simulink model "UZ_EnDat_be4_optimizing_agaib"  (R2023b)
settings: Solver=FixedStepDiscrete  StartTime=0  StopTime=0.002  RelTol=1e-3
model workspace (MAT data in the model file):
  Select = 0
libraries: hdlsllib x750, simulink x19, simulink_extras x4
(part 7 of 9)

== system UZ_EnDat_be4_optimizing_agaib/UZ_ENDAT/ManualSerialize/padder/nibblepadding22/padding1 ==
  in : Inport
  Bit Shift2 : hdlsllib/Logic and Bit Operations/Bit Shift  mode=Shift Right Logical  N=1
  Bit Slice2 : hdlsllib/Logic and Bit Operations/Bit Slice  lidx=0  ridx=0
  Data Type Conversion2 : DataTypeConversion  OutDataTypeStr=boolean  RndMeth=Nearest  SaturateOnIntegerOverflow=off
  Switch2 : Switch  Criteria=u2 > Threshold  SaturateOnIntegerOverflow=off  InputSameDT=off
  out : Outport
  wires:
  in/1 -> Bit Shift2/1, Switch2/1, Bit Slice2/1
  Bit Shift2/1 -> Switch2/3
  Data Type Conversion2/1 -> Switch2/2
  Bit Slice2/1 -> Data Type Conversion2/1
  Switch2/1 -> out/1

== system UZ_EnDat_be4_optimizing_agaib/UZ_ENDAT/ManualSerialize/padder/nibblepadding22/padding2 ==
  in : Inport
  Bit Shift2 : hdlsllib/Logic and Bit Operations/Bit Shift  mode=Shift Right Logical  N=1
  Bit Slice2 : hdlsllib/Logic and Bit Operations/Bit Slice  lidx=0  ridx=0
  Data Type Conversion2 : DataTypeConversion  OutDataTypeStr=boolean  RndMeth=Nearest  SaturateOnIntegerOverflow=off
  Switch2 : Switch  Criteria=u2 > Threshold  SaturateOnIntegerOverflow=off  InputSameDT=off
  out : Outport
  wires:
  in/1 -> Bit Shift2/1, Switch2/1, Bit Slice2/1
  Bit Shift2/1 -> Switch2/3
  Data Type Conversion2/1 -> Switch2/2
  Bit Slice2/1 -> Data Type Conversion2/1
  Switch2/1 -> out/1

== system UZ_EnDat_be4_optimizing_agaib/UZ_ENDAT/ManualSerialize/padder/nibblepadding22/padding3 ==
  in : Inport
  Bit Shift2 : hdlsllib/Logic and Bit Operations/Bit Shift  mode=Shift Right Logical  N=1
  Bit Slice2 : hdlsllib/Logic and Bit Operations/Bit Slice  lidx=0  ridx=0
  Data Type Conversion2 : DataTypeConversion  OutDataTypeStr=boolean  RndMeth=Nearest  SaturateOnIntegerOverflow=off
  Switch2 : Switch  Criteria=u2 > Threshold  SaturateOnIntegerOverflow=off  InputSameDT=off
  out : Outport
  wires:
  in/1 -> Bit Shift2/1, Switch2/1, Bit Slice2/1
  Bit Shift2/1 -> Switch2/3
  Data Type Conversion2/1 -> Switch2/2
  Bit Slice2/1 -> Data Type Conversion2/1
  Switch2/1 -> out/1

== system UZ_EnDat_be4_optimizing_agaib/UZ_ENDAT/ManualSerialize/padder/nibblepadding23/padding ==
  in : Inport
  Bit Shift2 : hdlsllib/Logic and Bit Operations/Bit Shift  mode=Shift Right Logical  N=1
  Bit Slice2 : hdlsllib/Logic and Bit Operations/Bit Slice  lidx=0  ridx=0
  Data Type Conversion2 : DataTypeConversion  OutDataTypeStr=boolean  RndMeth=Nearest  SaturateOnIntegerOverflow=off
  Switch2 : Switch  Criteria=u2 > Threshold  SaturateOnIntegerOverflow=off  InputSameDT=off
  out : Outport
  wires:
  in/1 -> Bit Shift2/1, Switch2/1, Bit Slice2/1
  Bit Shift2/1 -> Switch2/3
  Data Type Conversion2/1 -> Switch2/2
  Bit Slice2/1 -> Data Type Conversion2/1
  Switch2/1 -> out/1

== system UZ_EnDat_be4_optimizing_agaib/UZ_ENDAT/ManualSerialize/padder/nibblepadding23/padding1 ==
  in : Inport
  Bit Shift2 : hdlsllib/Logic and Bit Operations/Bit Shift  mode=Shift Right Logical  N=1
  Bit Slice2 : hdlsllib/Logic and Bit Operations/Bit Slice  lidx=0  ridx=0
  Data Type Conversion2 : DataTypeConversion  OutDataTypeStr=boolean  RndMeth=Nearest  SaturateOnIntegerOverflow=off
  Switch2 : Switch  Criteria=u2 > Threshold  SaturateOnIntegerOverflow=off  InputSameDT=off
  out : Outport
  wires:
  in/1 -> Bit Shift2/1, Switch2/1, Bit Slice2/1
  Bit Shift2/1 -> Switch2/3
  Data Type Conversion2/1 -> Switch2/2
  Bit Slice2/1 -> Data Type Conversion2/1
  Switch2/1 -> out/1

== system UZ_EnDat_be4_optimizing_agaib/UZ_ENDAT/ManualSerialize/padder/nibblepadding23/padding2 ==
  in : Inport
  Bit Shift2 : hdlsllib/Logic and Bit Operations/Bit Shift  mode=Shift Right Logical  N=1
  Bit Slice2 : hdlsllib/Logic and Bit Operations/Bit Slice  lidx=0  ridx=0
  Data Type Conversion2 : DataTypeConversion  OutDataTypeStr=boolean  RndMeth=Nearest  SaturateOnIntegerOverflow=off
  Switch2 : Switch  Criteria=u2 > Threshold  SaturateOnIntegerOverflow=off  InputSameDT=off
  out : Outport
  wires:
  in/1 -> Bit Shift2/1, Switch2/1, Bit Slice2/1
  Bit Shift2/1 -> Switch2/3
  Data Type Conversion2/1 -> Switch2/2
  Bit Slice2/1 -> Data Type Conversion2/1
  Switch2/1 -> out/1

== system UZ_EnDat_be4_optimizing_agaib/UZ_ENDAT/ManualSerialize/padder/nibblepadding23/padding3 ==
  in : Inport
  Bit Shift2 : hdlsllib/Logic and Bit Operations/Bit Shift  mode=Shift Right Logical  N=1
  Bit Slice2 : hdlsllib/Logic and Bit Operations/Bit Slice  lidx=0  ridx=0
  Data Type Conversion2 : DataTypeConversion  OutDataTypeStr=boolean  RndMeth=Nearest  SaturateOnIntegerOverflow=off
  Switch2 : Switch  Criteria=u2 > Threshold  SaturateOnIntegerOverflow=off  InputSameDT=off
  out : Outport
  wires:
  in/1 -> Bit Shift2/1, Switch2/1, Bit Slice2/1
  Bit Shift2/1 -> Switch2/3
  Data Type Conversion2/1 -> Switch2/2
  Bit Slice2/1 -> Data Type Conversion2/1
  Switch2/1 -> out/1

== system UZ_EnDat_be4_optimizing_agaib/UZ_ENDAT/ManualSerialize/padder/nibblepadding24/padding ==
  in : Inport
  Bit Shift2 : hdlsllib/Logic and Bit Operations/Bit Shift  mode=Shift Right Logical  N=1
  Bit Slice2 : hdlsllib/Logic and Bit Operations/Bit Slice  lidx=0  ridx=0
  Data Type Conversion2 : DataTypeConversion  OutDataTypeStr=boolean  RndMeth=Nearest  SaturateOnIntegerOverflow=off
  Switch2 : Switch  Criteria=u2 > Threshold  SaturateOnIntegerOverflow=off  InputSameDT=off
  out : Outport
  wires:
  in/1 -> Bit Shift2/1, Switch2/1, Bit Slice2/1
  Bit Shift2/1 -> Switch2/3
  Data Type Conversion2/1 -> Switch2/2
  Bit Slice2/1 -> Data Type Conversion2/1
  Switch2/1 -> out/1

== system UZ_EnDat_be4_optimizing_agaib/UZ_ENDAT/ManualSerialize/padder/nibblepadding24/padding1 ==
  in : Inport
  Bit Shift2 : hdlsllib/Logic and Bit Operations/Bit Shift  mode=Shift Right Logical  N=1
  Bit Slice2 : hdlsllib/Logic and Bit Operations/Bit Slice  lidx=0  ridx=0
  Data Type Conversion2 : DataTypeConversion  OutDataTypeStr=boolean  RndMeth=Nearest  SaturateOnIntegerOverflow=off
  Switch2 : Switch  Criteria=u2 > Threshold  SaturateOnIntegerOverflow=off  InputSameDT=off
  out : Outport
  wires:
  in/1 -> Bit Shift2/1, Switch2/1, Bit Slice2/1
  Bit Shift2/1 -> Switch2/3
  Data Type Conversion2/1 -> Switch2/2
  Bit Slice2/1 -> Data Type Conversion2/1
  Switch2/1 -> out/1

== system UZ_EnDat_be4_optimizing_agaib/UZ_ENDAT/ManualSerialize/padder/nibblepadding24/padding2 ==
  in : Inport
  Bit Shift2 : hdlsllib/Logic and Bit Operations/Bit Shift  mode=Shift Right Logical  N=1
  Bit Slice2 : hdlsllib/Logic and Bit Operations/Bit Slice  lidx=0  ridx=0
  Data Type Conversion2 : DataTypeConversion  OutDataTypeStr=boolean  RndMeth=Nearest  SaturateOnIntegerOverflow=off
  Switch2 : Switch  Criteria=u2 > Threshold  SaturateOnIntegerOverflow=off  InputSameDT=off
  out : Outport
  wires:
  in/1 -> Bit Shift2/1, Switch2/1, Bit Slice2/1
  Bit Shift2/1 -> Switch2/3
  Data Type Conversion2/1 -> Switch2/2
  Bit Slice2/1 -> Data Type Conversion2/1
  Switch2/1 -> out/1

== system UZ_EnDat_be4_optimizing_agaib/UZ_ENDAT/ManualSerialize/padder/nibblepadding24/padding3 ==
  in : Inport
  Bit Shift2 : hdlsllib/Logic and Bit Operations/Bit Shift  mode=Shift Right Logical  N=1
  Bit Slice2 : hdlsllib/Logic and Bit Operations/Bit Slice  lidx=0  ridx=0
  Data Type Conversion2 : DataTypeConversion  OutDataTypeStr=boolean  RndMeth=Nearest  SaturateOnIntegerOverflow=off
  Switch2 : Switch  Criteria=u2 > Threshold  SaturateOnIntegerOverflow=off  InputSameDT=off
  out : Outport
  wires:
  in/1 -> Bit Shift2/1, Switch2/1, Bit Slice2/1
  Bit Shift2/1 -> Switch2/3
  Data Type Conversion2/1 -> Switch2/2
  Bit Slice2/1 -> Data Type Conversion2/1
  Switch2/1 -> out/1

== system UZ_EnDat_be4_optimizing_agaib/UZ_ENDAT/ManualSerialize/padder/nibblepadding25/padding ==
  in : Inport
  Bit Shift2 : hdlsllib/Logic and Bit Operations/Bit Shift  mode=Shift Right Logical  N=1
  Bit Slice2 : hdlsllib/Logic and Bit Operations/Bit Slice  lidx=0  ridx=0
  Data Type Conversion2 : DataTypeConversion  OutDataTypeStr=boolean  RndMeth=Nearest  SaturateOnIntegerOverflow=off
  Switch2 : Switch  Criteria=u2 > Threshold  SaturateOnIntegerOverflow=off  InputSameDT=off
  out : Outport
  wires:
  in/1 -> Bit Shift2/1, Switch2/1, Bit Slice2/1
  Bit Shift2/1 -> Switch2/3
  Data Type Conversion2/1 -> Switch2/2
  Bit Slice2/1 -> Data Type Conversion2/1
  Switch2/1 -> out/1

== system UZ_EnDat_be4_optimizing_agaib/UZ_ENDAT/ManualSerialize/padder/nibblepadding25/padding1 ==
  in : Inport
  Bit Shift2 : hdlsllib/Logic and Bit Operations/Bit Shift  mode=Shift Right Logical  N=1
  Bit Slice2 : hdlsllib/Logic and Bit Operations/Bit Slice  lidx=0  ridx=0
  Data Type Conversion2 : DataTypeConversion  OutDataTypeStr=boolean  RndMeth=Nearest  SaturateOnIntegerOverflow=off
  Switch2 : Switch  Criteria=u2 > Threshold  SaturateOnIntegerOverflow=off  InputSameDT=off
  out : Outport
  wires:
  in/1 -> Bit Shift2/1, Switch2/1, Bit Slice2/1
  Bit Shift2/1 -> Switch2/3
  Data Type Conversion2/1 -> Switch2/2
  Bit Slice2/1 -> Data Type Conversion2/1
  Switch2/1 -> out/1

== system UZ_EnDat_be4_optimizing_agaib/UZ_ENDAT/ManualSerialize/padder/nibblepadding25/padding2 ==
  in : Inport
  Bit Shift2 : hdlsllib/Logic and Bit Operations/Bit Shift  mode=Shift Right Logical  N=1
  Bit Slice2 : hdlsllib/Logic and Bit Operations/Bit Slice  lidx=0  ridx=0
  Data Type Conversion2 : DataTypeConversion  OutDataTypeStr=boolean  RndMeth=Nearest  SaturateOnIntegerOverflow=off
  Switch2 : Switch  Criteria=u2 > Threshold  SaturateOnIntegerOverflow=off  InputSameDT=off
  out : Outport
  wires:
  in/1 -> Bit Shift2/1, Switch2/1, Bit Slice2/1
  Bit Shift2/1 -> Switch2/3
  Data Type Conversion2/1 -> Switch2/2
  Bit Slice2/1 -> Data Type Conversion2/1
  Switch2/1 -> out/1

== system UZ_EnDat_be4_optimizing_agaib/UZ_ENDAT/ManualSerialize/padder/nibblepadding25/padding3 ==
  in : Inport
  Bit Shift2 : hdlsllib/Logic and Bit Operations/Bit Shift  mode=Shift Right Logical  N=1
  Bit Slice2 : hdlsllib/Logic and Bit Operations/Bit Slice  lidx=0  ridx=0
  Data Type Conversion2 : DataTypeConversion  OutDataTypeStr=boolean  RndMeth=Nearest  SaturateOnIntegerOverflow=off
  Switch2 : Switch  Criteria=u2 > Threshold  SaturateOnIntegerOverflow=off  InputSameDT=off
  out : Outport
  wires:
  in/1 -> Bit Shift2/1, Switch2/1, Bit Slice2/1
  Bit Shift2/1 -> Switch2/3
  Data Type Conversion2/1 -> Switch2/2
  Bit Slice2/1 -> Data Type Conversion2/1
  Switch2/1 -> out/1

== system UZ_EnDat_be4_optimizing_agaib/UZ_ENDAT/ManualSerialize/padder/nibblepadding26/padding ==
  in : Inport
  Bit Shift2 : hdlsllib/Logic and Bit Operations/Bit Shift  mode=Shift Right Logical  N=1
  Bit Slice2 : hdlsllib/Logic and Bit Operations/Bit Slice  lidx=0  ridx=0
  Data Type Conversion2 : DataTypeConversion  OutDataTypeStr=boolean  RndMeth=Nearest  SaturateOnIntegerOverflow=off
  Switch2 : Switch  Criteria=u2 > Threshold  SaturateOnIntegerOverflow=off  InputSameDT=off
  out : Outport
  wires:
  in/1 -> Bit Shift2/1, Switch2/1, Bit Slice2/1
  Bit Shift2/1 -> Switch2/3
  Data Type Conversion2/1 -> Switch2/2
  Bit Slice2/1 -> Data Type Conversion2/1
  Switch2/1 -> out/1

== system UZ_EnDat_be4_optimizing_agaib/UZ_ENDAT/ManualSerialize/padder/nibblepadding26/padding1 ==
  in : Inport
  Bit Shift2 : hdlsllib/Logic and Bit Operations/Bit Shift  mode=Shift Right Logical  N=1
  Bit Slice2 : hdlsllib/Logic and Bit Operations/Bit Slice  lidx=0  ridx=0
  Data Type Conversion2 : DataTypeConversion  OutDataTypeStr=boolean  RndMeth=Nearest  SaturateOnIntegerOverflow=off
  Switch2 : Switch  Criteria=u2 > Threshold  SaturateOnIntegerOverflow=off  InputSameDT=off
  out : Outport
  wires:
  in/1 -> Bit Shift2/1, Switch2/1, Bit Slice2/1
  Bit Shift2/1 -> Switch2/3
  Data Type Conversion2/1 -> Switch2/2
  Bit Slice2/1 -> Data Type Conversion2/1
  Switch2/1 -> out/1

== system UZ_EnDat_be4_optimizing_agaib/UZ_ENDAT/ManualSerialize/padder/nibblepadding26/padding2 ==
  in : Inport
  Bit Shift2 : hdlsllib/Logic and Bit Operations/Bit Shift  mode=Shift Right Logical  N=1
  Bit Slice2 : hdlsllib/Logic and Bit Operations/Bit Slice  lidx=0  ridx=0
  Data Type Conversion2 : DataTypeConversion  OutDataTypeStr=boolean  RndMeth=Nearest  SaturateOnIntegerOverflow=off
  Switch2 : Switch  Criteria=u2 > Threshold  SaturateOnIntegerOverflow=off  InputSameDT=off
  out : Outport
  wires:
  in/1 -> Bit Shift2/1, Switch2/1, Bit Slice2/1
  Bit Shift2/1 -> Switch2/3
  Data Type Conversion2/1 -> Switch2/2
  Bit Slice2/1 -> Data Type Conversion2/1
  Switch2/1 -> out/1

== system UZ_EnDat_be4_optimizing_agaib/UZ_ENDAT/ManualSerialize/padder/nibblepadding26/padding3 ==
  in : Inport
  Bit Shift2 : hdlsllib/Logic and Bit Operations/Bit Shift  mode=Shift Right Logical  N=1
  Bit Slice2 : hdlsllib/Logic and Bit Operations/Bit Slice  lidx=0  ridx=0
  Data Type Conversion2 : DataTypeConversion  OutDataTypeStr=boolean  RndMeth=Nearest  SaturateOnIntegerOverflow=off
  Switch2 : Switch  Criteria=u2 > Threshold  SaturateOnIntegerOverflow=off  InputSameDT=off
  out : Outport
  wires:
  in/1 -> Bit Shift2/1, Switch2/1, Bit Slice2/1
  Bit Shift2/1 -> Switch2/3
  Data Type Conversion2/1 -> Switch2/2
  Bit Slice2/1 -> Data Type Conversion2/1
  Switch2/1 -> out/1

== system UZ_EnDat_be4_optimizing_agaib/UZ_ENDAT/ManualSerialize/padder/nibblepadding27/padding ==
  in : Inport
  Bit Shift2 : hdlsllib/Logic and Bit Operations/Bit Shift  mode=Shift Right Logical  N=1
  Bit Slice2 : hdlsllib/Logic and Bit Operations/Bit Slice  lidx=0  ridx=0
  Data Type Conversion2 : DataTypeConversion  OutDataTypeStr=boolean  RndMeth=Nearest  SaturateOnIntegerOverflow=off
  Switch2 : Switch  Criteria=u2 > Threshold  SaturateOnIntegerOverflow=off  InputSameDT=off
  out : Outport
  wires:
  in/1 -> Bit Shift2/1, Switch2/1, Bit Slice2/1
  Bit Shift2/1 -> Switch2/3
  Data Type Conversion2/1 -> Switch2/2
  Bit Slice2/1 -> Data Type Conversion2/1
  Switch2/1 -> out/1

== system UZ_EnDat_be4_optimizing_agaib/UZ_ENDAT/ManualSerialize/padder/nibblepadding27/padding1 ==
  in : Inport
  Bit Shift2 : hdlsllib/Logic and Bit Operations/Bit Shift  mode=Shift Right Logical  N=1
  Bit Slice2 : hdlsllib/Logic and Bit Operations/Bit Slice  lidx=0  ridx=0
  Data Type Conversion2 : DataTypeConversion  OutDataTypeStr=boolean  RndMeth=Nearest  SaturateOnIntegerOverflow=off
  Switch2 : Switch  Criteria=u2 > Threshold  SaturateOnIntegerOverflow=off  InputSameDT=off
  out : Outport
  wires:
  in/1 -> Bit Shift2/1, Switch2/1, Bit Slice2/1
  Bit Shift2/1 -> Switch2/3
  Data Type Conversion2/1 -> Switch2/2
  Bit Slice2/1 -> Data Type Conversion2/1
  Switch2/1 -> out/1

== system UZ_EnDat_be4_optimizing_agaib/UZ_ENDAT/ManualSerialize/padder/nibblepadding27/padding2 ==
  in : Inport
  Bit Shift2 : hdlsllib/Logic and Bit Operations/Bit Shift  mode=Shift Right Logical  N=1
  Bit Slice2 : hdlsllib/Logic and Bit Operations/Bit Slice  lidx=0  ridx=0
  Data Type Conversion2 : DataTypeConversion  OutDataTypeStr=boolean  RndMeth=Nearest  SaturateOnIntegerOverflow=off
  Switch2 : Switch  Criteria=u2 > Threshold  SaturateOnIntegerOverflow=off  InputSameDT=off
  out : Outport
  wires:
  in/1 -> Bit Shift2/1, Switch2/1, Bit Slice2/1
  Bit Shift2/1 -> Switch2/3
  Data Type Conversion2/1 -> Switch2/2
  Bit Slice2/1 -> Data Type Conversion2/1
  Switch2/1 -> out/1

== system UZ_EnDat_be4_optimizing_agaib/UZ_ENDAT/ManualSerialize/padder/nibblepadding27/padding3 ==
  in : Inport
  Bit Shift2 : hdlsllib/Logic and Bit Operations/Bit Shift  mode=Shift Right Logical  N=1
  Bit Slice2 : hdlsllib/Logic and Bit Operations/Bit Slice  lidx=0  ridx=0
  Data Type Conversion2 : DataTypeConversion  OutDataTypeStr=boolean  RndMeth=Nearest  SaturateOnIntegerOverflow=off
  Switch2 : Switch  Criteria=u2 > Threshold  SaturateOnIntegerOverflow=off  InputSameDT=off
  out : Outport
  wires:
  in/1 -> Bit Shift2/1, Switch2/1, Bit Slice2/1
  Bit Shift2/1 -> Switch2/3
  Data Type Conversion2/1 -> Switch2/2
  Bit Slice2/1 -> Data Type Conversion2/1
  Switch2/1 -> out/1

== system UZ_EnDat_be4_optimizing_agaib/UZ_ENDAT/ManualSerialize/padder/nibblepadding28/padding ==
  in : Inport
  Bit Shift2 : hdlsllib/Logic and Bit Operations/Bit Shift  mode=Shift Right Logical  N=1
  Bit Slice2 : hdlsllib/Logic and Bit Operations/Bit Slice  lidx=0  ridx=0
  Data Type Conversion2 : DataTypeConversion  OutDataTypeStr=boolean  RndMeth=Nearest  SaturateOnIntegerOverflow=off
  Switch2 : Switch  Criteria=u2 > Threshold  SaturateOnIntegerOverflow=off  InputSameDT=off
  out : Outport
  wires:
  in/1 -> Bit Shift2/1, Switch2/1, Bit Slice2/1
  Bit Shift2/1 -> Switch2/3
  Data Type Conversion2/1 -> Switch2/2
  Bit Slice2/1 -> Data Type Conversion2/1
  Switch2/1 -> out/1

== system UZ_EnDat_be4_optimizing_agaib/UZ_ENDAT/ManualSerialize/padder/nibblepadding28/padding1 ==
  in : Inport
  Bit Shift2 : hdlsllib/Logic and Bit Operations/Bit Shift  mode=Shift Right Logical  N=1
  Bit Slice2 : hdlsllib/Logic and Bit Operations/Bit Slice  lidx=0  ridx=0
  Data Type Conversion2 : DataTypeConversion  OutDataTypeStr=boolean  RndMeth=Nearest  SaturateOnIntegerOverflow=off
  Switch2 : Switch  Criteria=u2 > Threshold  SaturateOnIntegerOverflow=off  InputSameDT=off
  out : Outport
  wires:
  in/1 -> Bit Shift2/1, Switch2/1, Bit Slice2/1
  Bit Shift2/1 -> Switch2/3
  Data Type Conversion2/1 -> Switch2/2
  Bit Slice2/1 -> Data Type Conversion2/1
  Switch2/1 -> out/1

== system UZ_EnDat_be4_optimizing_agaib/UZ_ENDAT/ManualSerialize/padder/nibblepadding28/padding2 ==
  in : Inport
  Bit Shift2 : hdlsllib/Logic and Bit Operations/Bit Shift  mode=Shift Right Logical  N=1
  Bit Slice2 : hdlsllib/Logic and Bit Operations/Bit Slice  lidx=0  ridx=0
  Data Type Conversion2 : DataTypeConversion  OutDataTypeStr=boolean  RndMeth=Nearest  SaturateOnIntegerOverflow=off
  Switch2 : Switch  Criteria=u2 > Threshold  SaturateOnIntegerOverflow=off  InputSameDT=off
  out : Outport
  wires:
  in/1 -> Bit Shift2/1, Switch2/1, Bit Slice2/1
  Bit Shift2/1 -> Switch2/3
  Data Type Conversion2/1 -> Switch2/2
  Bit Slice2/1 -> Data Type Conversion2/1
  Switch2/1 -> out/1

== system UZ_EnDat_be4_optimizing_agaib/UZ_ENDAT/ManualSerialize/padder/nibblepadding28/padding3 ==
  in : Inport
  Bit Shift2 : hdlsllib/Logic and Bit Operations/Bit Shift  mode=Shift Right Logical  N=1
  Bit Slice2 : hdlsllib/Logic and Bit Operations/Bit Slice  lidx=0  ridx=0
  Data Type Conversion2 : DataTypeConversion  OutDataTypeStr=boolean  RndMeth=Nearest  SaturateOnIntegerOverflow=off
  Switch2 : Switch  Criteria=u2 > Threshold  SaturateOnIntegerOverflow=off  InputSameDT=off
  out : Outport
  wires:
  in/1 -> Bit Shift2/1, Switch2/1, Bit Slice2/1
  Bit Shift2/1 -> Switch2/3
  Data Type Conversion2/1 -> Switch2/2
  Bit Slice2/1 -> Data Type Conversion2/1
  Switch2/1 -> out/1

== system UZ_EnDat_be4_optimizing_agaib/UZ_ENDAT/ManualSerialize/padder/nibblepadding29/padding ==
  in : Inport
  Bit Shift2 : hdlsllib/Logic and Bit Operations/Bit Shift  mode=Shift Right Logical  N=1
  Bit Slice2 : hdlsllib/Logic and Bit Operations/Bit Slice  lidx=0  ridx=0
  Data Type Conversion2 : DataTypeConversion  OutDataTypeStr=boolean  RndMeth=Nearest  SaturateOnIntegerOverflow=off
  Switch2 : Switch  Criteria=u2 > Threshold  SaturateOnIntegerOverflow=off  InputSameDT=off
  out : Outport
  wires:
  in/1 -> Bit Shift2/1, Switch2/1, Bit Slice2/1
  Bit Shift2/1 -> Switch2/3
  Data Type Conversion2/1 -> Switch2/2
  Bit Slice2/1 -> Data Type Conversion2/1
  Switch2/1 -> out/1

== system UZ_EnDat_be4_optimizing_agaib/UZ_ENDAT/ManualSerialize/padder/nibblepadding29/padding1 ==
  in : Inport
  Bit Shift2 : hdlsllib/Logic and Bit Operations/Bit Shift  mode=Shift Right Logical  N=1
  Bit Slice2 : hdlsllib/Logic and Bit Operations/Bit Slice  lidx=0  ridx=0
  Data Type Conversion2 : DataTypeConversion  OutDataTypeStr=boolean  RndMeth=Nearest  SaturateOnIntegerOverflow=off
  Switch2 : Switch  Criteria=u2 > Threshold  SaturateOnIntegerOverflow=off  InputSameDT=off
  out : Outport
  wires:
  in/1 -> Bit Shift2/1, Switch2/1, Bit Slice2/1
  Bit Shift2/1 -> Switch2/3
  Data Type Conversion2/1 -> Switch2/2
  Bit Slice2/1 -> Data Type Conversion2/1
  Switch2/1 -> out/1

== system UZ_EnDat_be4_optimizing_agaib/UZ_ENDAT/ManualSerialize/padder/nibblepadding29/padding2 ==
  in : Inport
  Bit Shift2 : hdlsllib/Logic and Bit Operations/Bit Shift  mode=Shift Right Logical  N=1
  Bit Slice2 : hdlsllib/Logic and Bit Operations/Bit Slice  lidx=0  ridx=0
  Data Type Conversion2 : DataTypeConversion  OutDataTypeStr=boolean  RndMeth=Nearest  SaturateOnIntegerOverflow=off
  Switch2 : Switch  Criteria=u2 > Threshold  SaturateOnIntegerOverflow=off  InputSameDT=off
  out : Outport
  wires:
  in/1 -> Bit Shift2/1, Switch2/1, Bit Slice2/1
  Bit Shift2/1 -> Switch2/3
  Data Type Conversion2/1 -> Switch2/2
  Bit Slice2/1 -> Data Type Conversion2/1
  Switch2/1 -> out/1

== system UZ_EnDat_be4_optimizing_agaib/UZ_ENDAT/ManualSerialize/padder/nibblepadding29/padding3 ==
  in : Inport
  Bit Shift2 : hdlsllib/Logic and Bit Operations/Bit Shift  mode=Shift Right Logical  N=1
  Bit Slice2 : hdlsllib/Logic and Bit Operations/Bit Slice  lidx=0  ridx=0
  Data Type Conversion2 : DataTypeConversion  OutDataTypeStr=boolean  RndMeth=Nearest  SaturateOnIntegerOverflow=off
  Switch2 : Switch  Criteria=u2 > Threshold  SaturateOnIntegerOverflow=off  InputSameDT=off
  out : Outport
  wires:
  in/1 -> Bit Shift2/1, Switch2/1, Bit Slice2/1
  Bit Shift2/1 -> Switch2/3
  Data Type Conversion2/1 -> Switch2/2
  Bit Slice2/1 -> Data Type Conversion2/1
  Switch2/1 -> out/1

== system UZ_EnDat_be4_optimizing_agaib/UZ_ENDAT/ManualSerialize/padder/nibblepadding3/padding ==
  in : Inport
  Bit Shift2 : hdlsllib/Logic and Bit Operations/Bit Shift  mode=Shift Right Logical  N=1
  Bit Slice2 : hdlsllib/Logic and Bit Operations/Bit Slice  lidx=0  ridx=0
  Data Type Conversion2 : DataTypeConversion  OutDataTypeStr=boolean  RndMeth=Nearest  SaturateOnIntegerOverflow=off
  Switch2 : Switch  Criteria=u2 > Threshold  SaturateOnIntegerOverflow=off  InputSameDT=off
  out : Outport
  wires:
  in/1 -> Bit Shift2/1, Switch2/1, Bit Slice2/1
  Bit Shift2/1 -> Switch2/3
  Data Type Conversion2/1 -> Switch2/2
  Bit Slice2/1 -> Data Type Conversion2/1
  Switch2/1 -> out/1

== system UZ_EnDat_be4_optimizing_agaib/UZ_ENDAT/ManualSerialize/padder/nibblepadding3/padding1 ==
  in : Inport
  Bit Shift2 : hdlsllib/Logic and Bit Operations/Bit Shift  mode=Shift Right Logical  N=1
  Bit Slice2 : hdlsllib/Logic and Bit Operations/Bit Slice  lidx=0  ridx=0
  Data Type Conversion2 : DataTypeConversion  OutDataTypeStr=boolean  RndMeth=Nearest  SaturateOnIntegerOverflow=off
  Switch2 : Switch  Criteria=u2 > Threshold  SaturateOnIntegerOverflow=off  InputSameDT=off
  out : Outport
  wires:
  in/1 -> Bit Shift2/1, Switch2/1, Bit Slice2/1
  Bit Shift2/1 -> Switch2/3
  Data Type Conversion2/1 -> Switch2/2
  Bit Slice2/1 -> Data Type Conversion2/1
  Switch2/1 -> out/1

== system UZ_EnDat_be4_optimizing_agaib/UZ_ENDAT/ManualSerialize/padder/nibblepadding3/padding2 ==
  in : Inport
  Bit Shift2 : hdlsllib/Logic and Bit Operations/Bit Shift  mode=Shift Right Logical  N=1
  Bit Slice2 : hdlsllib/Logic and Bit Operations/Bit Slice  lidx=0  ridx=0
  Data Type Conversion2 : DataTypeConversion  OutDataTypeStr=boolean  RndMeth=Nearest  SaturateOnIntegerOverflow=off
  Switch2 : Switch  Criteria=u2 > Threshold  SaturateOnIntegerOverflow=off  InputSameDT=off
  out : Outport
  wires:
  in/1 -> Bit Shift2/1, Switch2/1, Bit Slice2/1
  Bit Shift2/1 -> Switch2/3
  Data Type Conversion2/1 -> Switch2/2
  Bit Slice2/1 -> Data Type Conversion2/1
  Switch2/1 -> out/1

== system UZ_EnDat_be4_optimizing_agaib/UZ_ENDAT/ManualSerialize/padder/nibblepadding3/padding3 ==
  in : Inport
  Bit Shift2 : hdlsllib/Logic and Bit Operations/Bit Shift  mode=Shift Right Logical  N=1
  Bit Slice2 : hdlsllib/Logic and Bit Operations/Bit Slice  lidx=0  ridx=0
  Data Type Conversion2 : DataTypeConversion  OutDataTypeStr=boolean  RndMeth=Nearest  SaturateOnIntegerOverflow=off
  Switch2 : Switch  Criteria=u2 > Threshold  SaturateOnIntegerOverflow=off  InputSameDT=off
  out : Outport
  wires:
  in/1 -> Bit Shift2/1, Switch2/1, Bit Slice2/1
  Bit Shift2/1 -> Switch2/3
  Data Type Conversion2/1 -> Switch2/2
  Bit Slice2/1 -> Data Type Conversion2/1
  Switch2/1 -> out/1

== system UZ_EnDat_be4_optimizing_agaib/UZ_ENDAT/ManualSerialize/padder/nibblepadding30/padding ==
  in : Inport
  Bit Shift2 : hdlsllib/Logic and Bit Operations/Bit Shift  mode=Shift Right Logical  N=1
  Bit Slice2 : hdlsllib/Logic and Bit Operations/Bit Slice  lidx=0  ridx=0
  Data Type Conversion2 : DataTypeConversion  OutDataTypeStr=boolean  RndMeth=Nearest  SaturateOnIntegerOverflow=off
  Switch2 : Switch  Criteria=u2 > Threshold  SaturateOnIntegerOverflow=off  InputSameDT=off
  out : Outport
  wires:
  in/1 -> Bit Shift2/1, Switch2/1, Bit Slice2/1
  Bit Shift2/1 -> Switch2/3
  Data Type Conversion2/1 -> Switch2/2
  Bit Slice2/1 -> Data Type Conversion2/1
  Switch2/1 -> out/1

== system UZ_EnDat_be4_optimizing_agaib/UZ_ENDAT/ManualSerialize/padder/nibblepadding30/padding1 ==
  in : Inport
  Bit Shift2 : hdlsllib/Logic and Bit Operations/Bit Shift  mode=Shift Right Logical  N=1
  Bit Slice2 : hdlsllib/Logic and Bit Operations/Bit Slice  lidx=0  ridx=0
  Data Type Conversion2 : DataTypeConversion  OutDataTypeStr=boolean  RndMeth=Nearest  SaturateOnIntegerOverflow=off
  Switch2 : Switch  Criteria=u2 > Threshold  SaturateOnIntegerOverflow=off  InputSameDT=off
  out : Outport
  wires:
  in/1 -> Bit Shift2/1, Switch2/1, Bit Slice2/1
  Bit Shift2/1 -> Switch2/3
  Data Type Conversion2/1 -> Switch2/2
  Bit Slice2/1 -> Data Type Conversion2/1
  Switch2/1 -> out/1

== system UZ_EnDat_be4_optimizing_agaib/UZ_ENDAT/ManualSerialize/padder/nibblepadding30/padding2 ==
  in : Inport
  Bit Shift2 : hdlsllib/Logic and Bit Operations/Bit Shift  mode=Shift Right Logical  N=1
  Bit Slice2 : hdlsllib/Logic and Bit Operations/Bit Slice  lidx=0  ridx=0
  Data Type Conversion2 : DataTypeConversion  OutDataTypeStr=boolean  RndMeth=Nearest  SaturateOnIntegerOverflow=off
  Switch2 : Switch  Criteria=u2 > Threshold  SaturateOnIntegerOverflow=off  InputSameDT=off
  out : Outport
  wires:
  in/1 -> Bit Shift2/1, Switch2/1, Bit Slice2/1
  Bit Shift2/1 -> Switch2/3
  Data Type Conversion2/1 -> Switch2/2
  Bit Slice2/1 -> Data Type Conversion2/1
  Switch2/1 -> out/1

== system UZ_EnDat_be4_optimizing_agaib/UZ_ENDAT/ManualSerialize/padder/nibblepadding30/padding3 ==
  in : Inport
  Bit Shift2 : hdlsllib/Logic and Bit Operations/Bit Shift  mode=Shift Right Logical  N=1
  Bit Slice2 : hdlsllib/Logic and Bit Operations/Bit Slice  lidx=0  ridx=0
  Data Type Conversion2 : DataTypeConversion  OutDataTypeStr=boolean  RndMeth=Nearest  SaturateOnIntegerOverflow=off
  Switch2 : Switch  Criteria=u2 > Threshold  SaturateOnIntegerOverflow=off  InputSameDT=off
  out : Outport
  wires:
  in/1 -> Bit Shift2/1, Switch2/1, Bit Slice2/1
  Bit Shift2/1 -> Switch2/3
  Data Type Conversion2/1 -> Switch2/2
  Bit Slice2/1 -> Data Type Conversion2/1
  Switch2/1 -> out/1

== system UZ_EnDat_be4_optimizing_agaib/UZ_ENDAT/ManualSerialize/padder/nibblepadding4/padding ==
  in : Inport
  Bit Shift2 : hdlsllib/Logic and Bit Operations/Bit Shift  mode=Shift Right Logical  N=1
  Bit Slice2 : hdlsllib/Logic and Bit Operations/Bit Slice  lidx=0  ridx=0
  Data Type Conversion2 : DataTypeConversion  OutDataTypeStr=boolean  RndMeth=Nearest  SaturateOnIntegerOverflow=off
  Switch2 : Switch  Criteria=u2 > Threshold  SaturateOnIntegerOverflow=off  InputSameDT=off
  out : Outport
  wires:
  in/1 -> Bit Shift2/1, Switch2/1, Bit Slice2/1
  Bit Shift2/1 -> Switch2/3
  Data Type Conversion2/1 -> Switch2/2
  Bit Slice2/1 -> Data Type Conversion2/1
  Switch2/1 -> out/1

== system UZ_EnDat_be4_optimizing_agaib/UZ_ENDAT/ManualSerialize/padder/nibblepadding4/padding1 ==
  in : Inport
  Bit Shift2 : hdlsllib/Logic and Bit Operations/Bit Shift  mode=Shift Right Logical  N=1
  Bit Slice2 : hdlsllib/Logic and Bit Operations/Bit Slice  lidx=0  ridx=0
  Data Type Conversion2 : DataTypeConversion  OutDataTypeStr=boolean  RndMeth=Nearest  SaturateOnIntegerOverflow=off
  Switch2 : Switch  Criteria=u2 > Threshold  SaturateOnIntegerOverflow=off  InputSameDT=off
  out : Outport
  wires:
  in/1 -> Bit Shift2/1, Switch2/1, Bit Slice2/1
  Bit Shift2/1 -> Switch2/3
  Data Type Conversion2/1 -> Switch2/2
  Bit Slice2/1 -> Data Type Conversion2/1
  Switch2/1 -> out/1

== system UZ_EnDat_be4_optimizing_agaib/UZ_ENDAT/ManualSerialize/padder/nibblepadding4/padding2 ==
  in : Inport
  Bit Shift2 : hdlsllib/Logic and Bit Operations/Bit Shift  mode=Shift Right Logical  N=1
  Bit Slice2 : hdlsllib/Logic and Bit Operations/Bit Slice  lidx=0  ridx=0
  Data Type Conversion2 : DataTypeConversion  OutDataTypeStr=boolean  RndMeth=Nearest  SaturateOnIntegerOverflow=off
  Switch2 : Switch  Criteria=u2 > Threshold  SaturateOnIntegerOverflow=off  InputSameDT=off
  out : Outport
  wires:
  in/1 -> Bit Shift2/1, Switch2/1, Bit Slice2/1
  Bit Shift2/1 -> Switch2/3
  Data Type Conversion2/1 -> Switch2/2
  Bit Slice2/1 -> Data Type Conversion2/1
  Switch2/1 -> out/1

== system UZ_EnDat_be4_optimizing_agaib/UZ_ENDAT/ManualSerialize/padder/nibblepadding4/padding3 ==
  in : Inport
  Bit Shift2 : hdlsllib/Logic and Bit Operations/Bit Shift  mode=Shift Right Logical  N=1
  Bit Slice2 : hdlsllib/Logic and Bit Operations/Bit Slice  lidx=0  ridx=0
  Data Type Conversion2 : DataTypeConversion  OutDataTypeStr=boolean  RndMeth=Nearest  SaturateOnIntegerOverflow=off
  Switch2 : Switch  Criteria=u2 > Threshold  SaturateOnIntegerOverflow=off  InputSameDT=off
  out : Outport
  wires:
  in/1 -> Bit Shift2/1, Switch2/1, Bit Slice2/1
  Bit Shift2/1 -> Switch2/3
  Data Type Conversion2/1 -> Switch2/2
  Bit Slice2/1 -> Data Type Conversion2/1
  Switch2/1 -> out/1

== system UZ_EnDat_be4_optimizing_agaib/UZ_ENDAT/ManualSerialize/padder/nibblepadding5/padding ==
  in : Inport
  Bit Shift2 : hdlsllib/Logic and Bit Operations/Bit Shift  mode=Shift Right Logical  N=1
  Bit Slice2 : hdlsllib/Logic and Bit Operations/Bit Slice  lidx=0  ridx=0
  Data Type Conversion2 : DataTypeConversion  OutDataTypeStr=boolean  RndMeth=Nearest  SaturateOnIntegerOverflow=off
  Switch2 : Switch  Criteria=u2 > Threshold  SaturateOnIntegerOverflow=off  InputSameDT=off
  out : Outport
  wires:
  in/1 -> Bit Shift2/1, Switch2/1, Bit Slice2/1
  Bit Shift2/1 -> Switch2/3
  Data Type Conversion2/1 -> Switch2/2
  Bit Slice2/1 -> Data Type Conversion2/1
  Switch2/1 -> out/1

== system UZ_EnDat_be4_optimizing_agaib/UZ_ENDAT/ManualSerialize/padder/nibblepadding5/padding1 ==
  in : Inport
  Bit Shift2 : hdlsllib/Logic and Bit Operations/Bit Shift  mode=Shift Right Logical  N=1
  Bit Slice2 : hdlsllib/Logic and Bit Operations/Bit Slice  lidx=0  ridx=0
  Data Type Conversion2 : DataTypeConversion  OutDataTypeStr=boolean  RndMeth=Nearest  SaturateOnIntegerOverflow=off
  Switch2 : Switch  Criteria=u2 > Threshold  SaturateOnIntegerOverflow=off  InputSameDT=off
  out : Outport
  wires:
  in/1 -> Bit Shift2/1, Switch2/1, Bit Slice2/1
  Bit Shift2/1 -> Switch2/3
  Data Type Conversion2/1 -> Switch2/2
  Bit Slice2/1 -> Data Type Conversion2/1
  Switch2/1 -> out/1

== system UZ_EnDat_be4_optimizing_agaib/UZ_ENDAT/ManualSerialize/padder/nibblepadding5/padding2 ==
  in : Inport
  Bit Shift2 : hdlsllib/Logic and Bit Operations/Bit Shift  mode=Shift Right Logical  N=1
  Bit Slice2 : hdlsllib/Logic and Bit Operations/Bit Slice  lidx=0  ridx=0
  Data Type Conversion2 : DataTypeConversion  OutDataTypeStr=boolean  RndMeth=Nearest  SaturateOnIntegerOverflow=off
  Switch2 : Switch  Criteria=u2 > Threshold  SaturateOnIntegerOverflow=off  InputSameDT=off
  out : Outport
  wires:
  in/1 -> Bit Shift2/1, Switch2/1, Bit Slice2/1
  Bit Shift2/1 -> Switch2/3
  Data Type Conversion2/1 -> Switch2/2
  Bit Slice2/1 -> Data Type Conversion2/1
  Switch2/1 -> out/1

== system UZ_EnDat_be4_optimizing_agaib/UZ_ENDAT/ManualSerialize/padder/nibblepadding5/padding3 ==
  in : Inport
  Bit Shift2 : hdlsllib/Logic and Bit Operations/Bit Shift  mode=Shift Right Logical  N=1
  Bit Slice2 : hdlsllib/Logic and Bit Operations/Bit Slice  lidx=0  ridx=0
  Data Type Conversion2 : DataTypeConversion  OutDataTypeStr=boolean  RndMeth=Nearest  SaturateOnIntegerOverflow=off
  Switch2 : Switch  Criteria=u2 > Threshold  SaturateOnIntegerOverflow=off  InputSameDT=off
  out : Outport
  wires:
  in/1 -> Bit Shift2/1, Switch2/1, Bit Slice2/1
  Bit Shift2/1 -> Switch2/3
  Data Type Conversion2/1 -> Switch2/2
  Bit Slice2/1 -> Data Type Conversion2/1
  Switch2/1 -> out/1

== system UZ_EnDat_be4_optimizing_agaib/UZ_ENDAT/ManualSerialize/padder/nibblepadding6/padding ==
  in : Inport
  Bit Shift2 : hdlsllib/Logic and Bit Operations/Bit Shift  mode=Shift Right Logical  N=1
  Bit Slice2 : hdlsllib/Logic and Bit Operations/Bit Slice  lidx=0  ridx=0
  Data Type Conversion2 : DataTypeConversion  OutDataTypeStr=boolean  RndMeth=Nearest  SaturateOnIntegerOverflow=off
  Switch2 : Switch  Criteria=u2 > Threshold  SaturateOnIntegerOverflow=off  InputSameDT=off
  out : Outport
  wires:
  in/1 -> Bit Shift2/1, Switch2/1, Bit Slice2/1
  Bit Shift2/1 -> Switch2/3
  Data Type Conversion2/1 -> Switch2/2
  Bit Slice2/1 -> Data Type Conversion2/1
  Switch2/1 -> out/1

== system UZ_EnDat_be4_optimizing_agaib/UZ_ENDAT/ManualSerialize/padder/nibblepadding6/padding1 ==
  in : Inport
  Bit Shift2 : hdlsllib/Logic and Bit Operations/Bit Shift  mode=Shift Right Logical  N=1
  Bit Slice2 : hdlsllib/Logic and Bit Operations/Bit Slice  lidx=0  ridx=0
  Data Type Conversion2 : DataTypeConversion  OutDataTypeStr=boolean  RndMeth=Nearest  SaturateOnIntegerOverflow=off
  Switch2 : Switch  Criteria=u2 > Threshold  SaturateOnIntegerOverflow=off  InputSameDT=off
  out : Outport
  wires:
  in/1 -> Bit Shift2/1, Switch2/1, Bit Slice2/1
  Bit Shift2/1 -> Switch2/3
  Data Type Conversion2/1 -> Switch2/2
  Bit Slice2/1 -> Data Type Conversion2/1
  Switch2/1 -> out/1

== system UZ_EnDat_be4_optimizing_agaib/UZ_ENDAT/ManualSerialize/padder/nibblepadding6/padding2 ==
  in : Inport
  Bit Shift2 : hdlsllib/Logic and Bit Operations/Bit Shift  mode=Shift Right Logical  N=1
  Bit Slice2 : hdlsllib/Logic and Bit Operations/Bit Slice  lidx=0  ridx=0
  Data Type Conversion2 : DataTypeConversion  OutDataTypeStr=boolean  RndMeth=Nearest  SaturateOnIntegerOverflow=off
  Switch2 : Switch  Criteria=u2 > Threshold  SaturateOnIntegerOverflow=off  InputSameDT=off
  out : Outport
  wires:
  in/1 -> Bit Shift2/1, Switch2/1, Bit Slice2/1
  Bit Shift2/1 -> Switch2/3
  Data Type Conversion2/1 -> Switch2/2
  Bit Slice2/1 -> Data Type Conversion2/1
  Switch2/1 -> out/1

== system UZ_EnDat_be4_optimizing_agaib/UZ_ENDAT/ManualSerialize/padder/nibblepadding6/padding3 ==
  in : Inport
  Bit Shift2 : hdlsllib/Logic and Bit Operations/Bit Shift  mode=Shift Right Logical  N=1
  Bit Slice2 : hdlsllib/Logic and Bit Operations/Bit Slice  lidx=0  ridx=0
  Data Type Conversion2 : DataTypeConversion  OutDataTypeStr=boolean  RndMeth=Nearest  SaturateOnIntegerOverflow=off
  Switch2 : Switch  Criteria=u2 > Threshold  SaturateOnIntegerOverflow=off  InputSameDT=off
  out : Outport
  wires:
  in/1 -> Bit Shift2/1, Switch2/1, Bit Slice2/1
  Bit Shift2/1 -> Switch2/3
  Data Type Conversion2/1 -> Switch2/2
  Bit Slice2/1 -> Data Type Conversion2/1
  Switch2/1 -> out/1

== system UZ_EnDat_be4_optimizing_agaib/UZ_ENDAT/ManualSerialize/padder/nibblepadding7/padding ==
  in : Inport
  Bit Shift2 : hdlsllib/Logic and Bit Operations/Bit Shift  mode=Shift Right Logical  N=1
  Bit Slice2 : hdlsllib/Logic and Bit Operations/Bit Slice  lidx=0  ridx=0
  Data Type Conversion2 : DataTypeConversion  OutDataTypeStr=boolean  RndMeth=Nearest  SaturateOnIntegerOverflow=off
  Switch2 : Switch  Criteria=u2 > Threshold  SaturateOnIntegerOverflow=off  InputSameDT=off
  out : Outport
  wires:
  in/1 -> Bit Shift2/1, Switch2/1, Bit Slice2/1
  Bit Shift2/1 -> Switch2/3
  Data Type Conversion2/1 -> Switch2/2
  Bit Slice2/1 -> Data Type Conversion2/1
  Switch2/1 -> out/1

== system UZ_EnDat_be4_optimizing_agaib/UZ_ENDAT/ManualSerialize/padder/nibblepadding7/padding1 ==
  in : Inport
  Bit Shift2 : hdlsllib/Logic and Bit Operations/Bit Shift  mode=Shift Right Logical  N=1
  Bit Slice2 : hdlsllib/Logic and Bit Operations/Bit Slice  lidx=0  ridx=0
  Data Type Conversion2 : DataTypeConversion  OutDataTypeStr=boolean  RndMeth=Nearest  SaturateOnIntegerOverflow=off
  Switch2 : Switch  Criteria=u2 > Threshold  SaturateOnIntegerOverflow=off  InputSameDT=off
  out : Outport
  wires:
  in/1 -> Bit Shift2/1, Switch2/1, Bit Slice2/1
  Bit Shift2/1 -> Switch2/3
  Data Type Conversion2/1 -> Switch2/2
  Bit Slice2/1 -> Data Type Conversion2/1
  Switch2/1 -> out/1

== system UZ_EnDat_be4_optimizing_agaib/UZ_ENDAT/ManualSerialize/padder/nibblepadding7/padding2 ==
  in : Inport
  Bit Shift2 : hdlsllib/Logic and Bit Operations/Bit Shift  mode=Shift Right Logical  N=1
  Bit Slice2 : hdlsllib/Logic and Bit Operations/Bit Slice  lidx=0  ridx=0
  Data Type Conversion2 : DataTypeConversion  OutDataTypeStr=boolean  RndMeth=Nearest  SaturateOnIntegerOverflow=off
  Switch2 : Switch  Criteria=u2 > Threshold  SaturateOnIntegerOverflow=off  InputSameDT=off
  out : Outport
  wires:
  in/1 -> Bit Shift2/1, Switch2/1, Bit Slice2/1
  Bit Shift2/1 -> Switch2/3
  Data Type Conversion2/1 -> Switch2/2
  Bit Slice2/1 -> Data Type Conversion2/1
  Switch2/1 -> out/1

== system UZ_EnDat_be4_optimizing_agaib/UZ_ENDAT/ManualSerialize/padder/nibblepadding7/padding3 ==
  in : Inport
  Bit Shift2 : hdlsllib/Logic and Bit Operations/Bit Shift  mode=Shift Right Logical  N=1
  Bit Slice2 : hdlsllib/Logic and Bit Operations/Bit Slice  lidx=0  ridx=0
  Data Type Conversion2 : DataTypeConversion  OutDataTypeStr=boolean  RndMeth=Nearest  SaturateOnIntegerOverflow=off
  Switch2 : Switch  Criteria=u2 > Threshold  SaturateOnIntegerOverflow=off  InputSameDT=off
  out : Outport
  wires:
  in/1 -> Bit Shift2/1, Switch2/1, Bit Slice2/1
  Bit Shift2/1 -> Switch2/3
  Data Type Conversion2/1 -> Switch2/2
  Bit Slice2/1 -> Data Type Conversion2/1
  Switch2/1 -> out/1

== system UZ_EnDat_be4_optimizing_agaib/UZ_ENDAT/ManualSerialize/padder/nibblepadding8/padding ==
  in : Inport
  Bit Shift2 : hdlsllib/Logic and Bit Operations/Bit Shift  mode=Shift Right Logical  N=1
  Bit Slice2 : hdlsllib/Logic and Bit Operations/Bit Slice  lidx=0  ridx=0
  Data Type Conversion2 : DataTypeConversion  OutDataTypeStr=boolean  RndMeth=Nearest  SaturateOnIntegerOverflow=off
  Switch2 : Switch  Criteria=u2 > Threshold  SaturateOnIntegerOverflow=off  InputSameDT=off
  out : Outport
  wires:
  in/1 -> Bit Shift2/1, Switch2/1, Bit Slice2/1
  Bit Shift2/1 -> Switch2/3
  Data Type Conversion2/1 -> Switch2/2
  Bit Slice2/1 -> Data Type Conversion2/1
  Switch2/1 -> out/1

== system UZ_EnDat_be4_optimizing_agaib/UZ_ENDAT/ManualSerialize/padder/nibblepadding8/padding1 ==
  in : Inport
  Bit Shift2 : hdlsllib/Logic and Bit Operations/Bit Shift  mode=Shift Right Logical  N=1
  Bit Slice2 : hdlsllib/Logic and Bit Operations/Bit Slice  lidx=0  ridx=0
  Data Type Conversion2 : DataTypeConversion  OutDataTypeStr=boolean  RndMeth=Nearest  SaturateOnIntegerOverflow=off
  Switch2 : Switch  Criteria=u2 > Threshold  SaturateOnIntegerOverflow=off  InputSameDT=off
  out : Outport
  wires:
  in/1 -> Bit Shift2/1, Switch2/1, Bit Slice2/1
  Bit Shift2/1 -> Switch2/3
  Data Type Conversion2/1 -> Switch2/2
  Bit Slice2/1 -> Data Type Conversion2/1
  Switch2/1 -> out/1

== system UZ_EnDat_be4_optimizing_agaib/UZ_ENDAT/ManualSerialize/padder/nibblepadding8/padding2 ==
  in : Inport
  Bit Shift2 : hdlsllib/Logic and Bit Operations/Bit Shift  mode=Shift Right Logical  N=1
  Bit Slice2 : hdlsllib/Logic and Bit Operations/Bit Slice  lidx=0  ridx=0
  Data Type Conversion2 : DataTypeConversion  OutDataTypeStr=boolean  RndMeth=Nearest  SaturateOnIntegerOverflow=off
  Switch2 : Switch  Criteria=u2 > Threshold  SaturateOnIntegerOverflow=off  InputSameDT=off
  out : Outport
  wires:
  in/1 -> Bit Shift2/1, Switch2/1, Bit Slice2/1
  Bit Shift2/1 -> Switch2/3
  Data Type Conversion2/1 -> Switch2/2
  Bit Slice2/1 -> Data Type Conversion2/1
  Switch2/1 -> out/1

== system UZ_EnDat_be4_optimizing_agaib/UZ_ENDAT/ManualSerialize/padder/nibblepadding8/padding3 ==
  in : Inport
  Bit Shift2 : hdlsllib/Logic and Bit Operations/Bit Shift  mode=Shift Right Logical  N=1
  Bit Slice2 : hdlsllib/Logic and Bit Operations/Bit Slice  lidx=0  ridx=0
  Data Type Conversion2 : DataTypeConversion  OutDataTypeStr=boolean  RndMeth=Nearest  SaturateOnIntegerOverflow=off
  Switch2 : Switch  Criteria=u2 > Threshold  SaturateOnIntegerOverflow=off  InputSameDT=off
  out : Outport
  wires:
  in/1 -> Bit Shift2/1, Switch2/1, Bit Slice2/1
  Bit Shift2/1 -> Switch2/3
  Data Type Conversion2/1 -> Switch2/2
  Bit Slice2/1 -> Data Type Conversion2/1
  Switch2/1 -> out/1

== system UZ_EnDat_be4_optimizing_agaib/UZ_ENDAT/ManualSerialize/padder/nibblepadding9/padding ==
  in : Inport
  Bit Shift2 : hdlsllib/Logic and Bit Operations/Bit Shift  mode=Shift Right Logical  N=1
  Bit Slice2 : hdlsllib/Logic and Bit Operations/Bit Slice  lidx=0  ridx=0
  Data Type Conversion2 : DataTypeConversion  OutDataTypeStr=boolean  RndMeth=Nearest  SaturateOnIntegerOverflow=off
  Switch2 : Switch  Criteria=u2 > Threshold  SaturateOnIntegerOverflow=off  InputSameDT=off
  out : Outport
  wires:
  in/1 -> Bit Shift2/1, Switch2/1, Bit Slice2/1
  Bit Shift2/1 -> Switch2/3
  Data Type Conversion2/1 -> Switch2/2
  Bit Slice2/1 -> Data Type Conversion2/1
  Switch2/1 -> out/1

== system UZ_EnDat_be4_optimizing_agaib/UZ_ENDAT/ManualSerialize/padder/nibblepadding9/padding1 ==
  in : Inport
  Bit Shift2 : hdlsllib/Logic and Bit Operations/Bit Shift  mode=Shift Right Logical  N=1
  Bit Slice2 : hdlsllib/Logic and Bit Operations/Bit Slice  lidx=0  ridx=0
  Data Type Conversion2 : DataTypeConversion  OutDataTypeStr=boolean  RndMeth=Nearest  SaturateOnIntegerOverflow=off
  Switch2 : Switch  Criteria=u2 > Threshold  SaturateOnIntegerOverflow=off  InputSameDT=off
  out : Outport
  wires:
  in/1 -> Bit Shift2/1, Switch2/1, Bit Slice2/1
  Bit Shift2/1 -> Switch2/3
  Data Type Conversion2/1 -> Switch2/2
  Bit Slice2/1 -> Data Type Conversion2/1
  Switch2/1 -> out/1

== system UZ_EnDat_be4_optimizing_agaib/UZ_ENDAT/ManualSerialize/padder/nibblepadding9/padding2 ==
  in : Inport
  Bit Shift2 : hdlsllib/Logic and Bit Operations/Bit Shift  mode=Shift Right Logical  N=1
  Bit Slice2 : hdlsllib/Logic and Bit Operations/Bit Slice  lidx=0  ridx=0
  Data Type Conversion2 : DataTypeConversion  OutDataTypeStr=boolean  RndMeth=Nearest  SaturateOnIntegerOverflow=off
  Switch2 : Switch  Criteria=u2 > Threshold  SaturateOnIntegerOverflow=off  InputSameDT=off
  out : Outport
  wires:
  in/1 -> Bit Shift2/1, Switch2/1, Bit Slice2/1
  Bit Shift2/1 -> Switch2/3
  Data Type Conversion2/1 -> Switch2/2
  Bit Slice2/1 -> Data Type Conversion2/1
  Switch2/1 -> out/1

== system UZ_EnDat_be4_optimizing_agaib/UZ_ENDAT/ManualSerialize/padder/nibblepadding9/padding3 ==
  in : Inport
  Bit Shift2 : hdlsllib/Logic and Bit Operations/Bit Shift  mode=Shift Right Logical  N=1
  Bit Slice2 : hdlsllib/Logic and Bit Operations/Bit Slice  lidx=0  ridx=0
  Data Type Conversion2 : DataTypeConversion  OutDataTypeStr=boolean  RndMeth=Nearest  SaturateOnIntegerOverflow=off
  Switch2 : Switch  Criteria=u2 > Threshold  SaturateOnIntegerOverflow=off  InputSameDT=off
  out : Outport
  wires:
  in/1 -> Bit Shift2/1, Switch2/1, Bit Slice2/1
  Bit Shift2/1 -> Switch2/3
  Data Type Conversion2/1 -> Switch2/2
  Bit Slice2/1 -> Data Type Conversion2/1
  Switch2/1 -> out/1

== system UZ_EnDat_be4_optimizing_agaib/UZ_ENDAT/ManualSerialize1/padder/nibblepadding1/padding ==
  in : Inport
  Bit Shift2 : hdlsllib/Logic and Bit Operations/Bit Shift  mode=Shift Right Logical  N=1
  Bit Slice2 : hdlsllib/Logic and Bit Operations/Bit Slice  lidx=0  ridx=0
  Data Type Conversion2 : DataTypeConversion  OutDataTypeStr=boolean  RndMeth=Nearest  SaturateOnIntegerOverflow=off
  Switch2 : Switch  Criteria=u2 > Threshold  SaturateOnIntegerOverflow=off  InputSameDT=off
  out : Outport
  wires:
  in/1 -> Bit Shift2/1, Switch2/1, Bit Slice2/1
  Bit Shift2/1 -> Switch2/3
  Data Type Conversion2/1 -> Switch2/2
  Bit Slice2/1 -> Data Type Conversion2/1
  Switch2/1 -> out/1

== system UZ_EnDat_be4_optimizing_agaib/UZ_ENDAT/ManualSerialize1/padder/nibblepadding1/padding1 ==
  in : Inport
  Bit Shift2 : hdlsllib/Logic and Bit Operations/Bit Shift  mode=Shift Right Logical  N=1
  Bit Slice2 : hdlsllib/Logic and Bit Operations/Bit Slice  lidx=0  ridx=0
  Data Type Conversion2 : DataTypeConversion  OutDataTypeStr=boolean  RndMeth=Nearest  SaturateOnIntegerOverflow=off
  Switch2 : Switch  Criteria=u2 > Threshold  SaturateOnIntegerOverflow=off  InputSameDT=off
  out : Outport
  wires:
  in/1 -> Bit Shift2/1, Switch2/1, Bit Slice2/1
  Bit Shift2/1 -> Switch2/3
  Data Type Conversion2/1 -> Switch2/2
  Bit Slice2/1 -> Data Type Conversion2/1
  Switch2/1 -> out/1

== system UZ_EnDat_be4_optimizing_agaib/UZ_ENDAT/ManualSerialize1/padder/nibblepadding1/padding2 ==
  in : Inport
  Bit Shift2 : hdlsllib/Logic and Bit Operations/Bit Shift  mode=Shift Right Logical  N=1
  Bit Slice2 : hdlsllib/Logic and Bit Operations/Bit Slice  lidx=0  ridx=0
  Data Type Conversion2 : DataTypeConversion  OutDataTypeStr=boolean  RndMeth=Nearest  SaturateOnIntegerOverflow=off
  Switch2 : Switch  Criteria=u2 > Threshold  SaturateOnIntegerOverflow=off  InputSameDT=off
  out : Outport
  wires:
  in/1 -> Bit Shift2/1, Switch2/1, Bit Slice2/1
  Bit Shift2/1 -> Switch2/3
  Data Type Conversion2/1 -> Switch2/2
  Bit Slice2/1 -> Data Type Conversion2/1
  Switch2/1 -> out/1

== system UZ_EnDat_be4_optimizing_agaib/UZ_ENDAT/ManualSerialize1/padder/nibblepadding1/padding3 ==
  in : Inport
  Bit Shift2 : hdlsllib/Logic and Bit Operations/Bit Shift  mode=Shift Right Logical  N=1
  Bit Slice2 : hdlsllib/Logic and Bit Operations/Bit Slice  lidx=0  ridx=0
  Data Type Conversion2 : DataTypeConversion  OutDataTypeStr=boolean  RndMeth=Nearest  SaturateOnIntegerOverflow=off
  Switch2 : Switch  Criteria=u2 > Threshold  SaturateOnIntegerOverflow=off  InputSameDT=off
  out : Outport
  wires:
  in/1 -> Bit Shift2/1, Switch2/1, Bit Slice2/1
  Bit Shift2/1 -> Switch2/3
  Data Type Conversion2/1 -> Switch2/2
  Bit Slice2/1 -> Data Type Conversion2/1
  Switch2/1 -> out/1

== system UZ_EnDat_be4_optimizing_agaib/UZ_ENDAT/ManualSerialize1/padder/nibblepadding10/padding ==
  in : Inport
  Bit Shift2 : hdlsllib/Logic and Bit Operations/Bit Shift  mode=Shift Right Logical  N=1
  Bit Slice2 : hdlsllib/Logic and Bit Operations/Bit Slice  lidx=0  ridx=0
  Data Type Conversion2 : DataTypeConversion  OutDataTypeStr=boolean  RndMeth=Nearest  SaturateOnIntegerOverflow=off
  Switch2 : Switch  Criteria=u2 > Threshold  SaturateOnIntegerOverflow=off  InputSameDT=off
  out : Outport
  wires:
  in/1 -> Bit Shift2/1, Switch2/1, Bit Slice2/1
  Bit Shift2/1 -> Switch2/3
  Data Type Conversion2/1 -> Switch2/2
  Bit Slice2/1 -> Data Type Conversion2/1
  Switch2/1 -> out/1

== system UZ_EnDat_be4_optimizing_agaib/UZ_ENDAT/ManualSerialize1/padder/nibblepadding10/padding1 ==
  in : Inport
  Bit Shift2 : hdlsllib/Logic and Bit Operations/Bit Shift  mode=Shift Right Logical  N=1
  Bit Slice2 : hdlsllib/Logic and Bit Operations/Bit Slice  lidx=0  ridx=0
  Data Type Conversion2 : DataTypeConversion  OutDataTypeStr=boolean  RndMeth=Nearest  SaturateOnIntegerOverflow=off
  Switch2 : Switch  Criteria=u2 > Threshold  SaturateOnIntegerOverflow=off  InputSameDT=off
  out : Outport
  wires:
  in/1 -> Bit Shift2/1, Switch2/1, Bit Slice2/1
  Bit Shift2/1 -> Switch2/3
  Data Type Conversion2/1 -> Switch2/2
  Bit Slice2/1 -> Data Type Conversion2/1
  Switch2/1 -> out/1

== system UZ_EnDat_be4_optimizing_agaib/UZ_ENDAT/ManualSerialize1/padder/nibblepadding10/padding2 ==
  in : Inport
  Bit Shift2 : hdlsllib/Logic and Bit Operations/Bit Shift  mode=Shift Right Logical  N=1
  Bit Slice2 : hdlsllib/Logic and Bit Operations/Bit Slice  lidx=0  ridx=0
  Data Type Conversion2 : DataTypeConversion  OutDataTypeStr=boolean  RndMeth=Nearest  SaturateOnIntegerOverflow=off
  Switch2 : Switch  Criteria=u2 > Threshold  SaturateOnIntegerOverflow=off  InputSameDT=off
  out : Outport
  wires:
  in/1 -> Bit Shift2/1, Switch2/1, Bit Slice2/1
  Bit Shift2/1 -> Switch2/3
  Data Type Conversion2/1 -> Switch2/2
  Bit Slice2/1 -> Data Type Conversion2/1
  Switch2/1 -> out/1

== system UZ_EnDat_be4_optimizing_agaib/UZ_ENDAT/ManualSerialize1/padder/nibblepadding10/padding3 ==
  in : Inport
  Bit Shift2 : hdlsllib/Logic and Bit Operations/Bit Shift  mode=Shift Right Logical  N=1
  Bit Slice2 : hdlsllib/Logic and Bit Operations/Bit Slice  lidx=0  ridx=0
  Data Type Conversion2 : DataTypeConversion  OutDataTypeStr=boolean  RndMeth=Nearest  SaturateOnIntegerOverflow=off
  Switch2 : Switch  Criteria=u2 > Threshold  SaturateOnIntegerOverflow=off  InputSameDT=off
  out : Outport
  wires:
  in/1 -> Bit Shift2/1, Switch2/1, Bit Slice2/1
  Bit Shift2/1 -> Switch2/3
  Data Type Conversion2/1 -> Switch2/2
  Bit Slice2/1 -> Data Type Conversion2/1
  Switch2/1 -> out/1
